simulink model "onolfihjsihjn"  (R2018b)
settings: Solver=FixedStepAuto  StartTime=0.0  StopTime=500  FixedStep=0.1  MaxStep=1E-3  RelTol=1e-3
values from neighbouring files (symbols this model uses):
  Ad = [1  0.1; 0  1]    [data_ver2.mat]    (also in data_ver3.mat = [1  0.5; 0  1]; just_running.m = sysd.A)
  bd = [0.005 0.1]    [data_ver2.mat]    (also in data_ver3.mat = [0.125 0.5]; just_running.m = sysd.B)
  SumoTs = block.DialogPrm(1).Data    [LeaderBlock.m]    (also in ObjectBlock.m; data_ver2.mat = 0.1; data_ver3.mat = 0.5; just_running.m = 0.5)
libraries: simulink x2
settings Model: Creator=HP  LastModifiedBy=HP

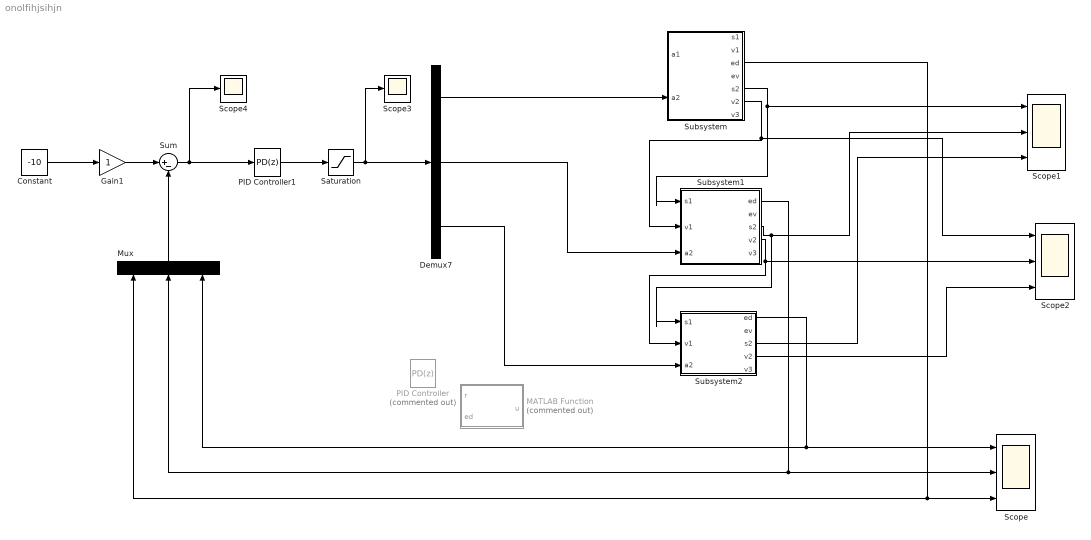
== system onolfihjsihjn ==
  Constant : Constant  Value=-10
  Demux7 : Demux  Outputs=3
  Gain1 : Gain
  MATLAB Function : MATLAB Function  Commented=on  TreatAsAtomicUnit=on
  Mux : Mux  Inputs=3
  PID Controller : simulink/Continuous/PID Controller  Commented=on  Controller=PD  Form=Parallel  TimeDomain=Discrete-time  SampleTime=-1  IntegratorMethod=Forward Euler  FilterMethod=Forward Euler  ControllerParametersSource=internal  P=0.1  I=1  D=1  UseFilter=off  N=1  TunerSelectOption=Transfer Function Based (PID Tuner App)  InitialConditionSource=internal  InitialConditionForIntegrator=0  InitialConditionForFilter=0  DifferentiatorICPrevScaledInput=0  ExternalReset=none  TrackingMode=off  Kt=1  LimitOutput=off  UpperSaturationLimit=inf  LowerSaturationLimit=-inf  LinearizeAsGain=on  AntiWindupMode=none  Kb=1  POutMin=[]  POutMax=[]  IOutMin=[]  IOutMax=[]  DOutMin=[]  DOutMax=[]  NOutMin=[]  NOutMax=[]  SumOutMin=[]  SumOutMax=[]  SaturationOutMin=[]  SaturationOutMax=[]  PParamMin=[]  PParamMax=[]  IParamMin=[]  IParamMax=[]  DParamMin=[]  DParamMax=[]  NParamMin=[]  NParamMax=[]  KbParamMin=[]  KbParamMax=[]  KtParamMin=[]  KtParamMax=[]  KbOutMin=[]  KbOutMax=[]  KtOutMin=[]  KtOutMax=[]  IntegratorOutMin=[]  IntegratorOutMax=[]  FilterOutMin=[]  FilterOutMax=[]  SumI1OutMin=[]  SumI1OutMax=[]  SumI2OutMin=[]  SumI2OutMax=[]  SumI3OutMin=[]  SumI3OutMax=[]  SumI4OutMin=[]  SumI4OutMax=[]  SumDOutMin=[]  SumDOutMax=[]  DifferentiatorOutMin=[]  DifferentiatorOutMax=[]  FilterDiffOutCoefMin=[]  FilterDiffOutCoefMax=[]  ReciprocalOutMin=[]  ReciprocalOutMax=[]  SumDenOutMin=[]  SumDenOutMax=[]  SumNumOutMin=[]  SumNumOutMax=[]  DivideOutMin=[]  DivideOutMax=[]  IntegratorContinuousStateAttributes=''  IntegratorStateMustResolveToSignalObject=off  IntegratorRTWStateStorageClass=Auto  FilterContinuousStateAttributes=''  FilterStateMustResolveToSignalObject=off  FilterRTWStateStorageClass=Auto  ParallelPVariant=InternalParameters  IdealPVariant=Disabled  IVariant=Disabled  DVariant=InternalParameters  IntegratorVariant=Disabled  SatVariant=Disabled  AWVariant=Disabled  PCopyVariant=Disabled  TRVariant=Disabled  FdbkBlocksVariant=Forward  IdealPFdbkVariant=Disabled  SatFdbkVariant=Disabled  DerivativeFilterVariant=Differentiator  NVariant=Passthrough  NCopyVariant=Disabled_SignalSpec  FilterICVariant=InternalICsDifferentiator  IntegratorICVariant=Disabled  ExternalResetVariant=Disabled  TRSumVariant=Passthrough  SumFdbkVariant=Disabled  SumVariant=Sum_PD
  PID Controller1 : simulink/Continuous/PID Controller  Controller=PD  Form=Parallel  TimeDomain=Discrete-time  SampleTime=-1  IntegratorMethod=Forward Euler  FilterMethod=Forward Euler  ControllerParametersSource=internal  P=0.1  I=1  D=0.8  UseFilter=off  N=1  TunerSelectOption=Transfer Function Based (PID Tuner App)  InitialConditionSource=internal  InitialConditionForIntegrator=0  InitialConditionForFilter=0  DifferentiatorICPrevScaledInput=0  ExternalReset=none  TrackingMode=off  Kt=1  LimitOutput=off  UpperSaturationLimit=inf  LowerSaturationLimit=-inf  LinearizeAsGain=on  AntiWindupMode=none  Kb=1  POutMin=[]  POutMax=[]  IOutMin=[]  IOutMax=[]  DOutMin=[]  DOutMax=[]  NOutMin=[]  NOutMax=[]  SumOutMin=[]  SumOutMax=[]  SaturationOutMin=[]  SaturationOutMax=[]  PParamMin=[]  PParamMax=[]  IParamMin=[]  IParamMax=[]  DParamMin=[]  DParamMax=[]  NParamMin=[]  NParamMax=[]  KbParamMin=[]  KbParamMax=[]  KtParamMin=[]  KtParamMax=[]  KbOutMin=[]  KbOutMax=[]  KtOutMin=[]  KtOutMax=[]  IntegratorOutMin=[]  IntegratorOutMax=[]  FilterOutMin=[]  FilterOutMax=[]  SumI1OutMin=[]  SumI1OutMax=[]  SumI2OutMin=[]  SumI2OutMax=[]  SumI3OutMin=[]  SumI3OutMax=[]  SumI4OutMin=[]  SumI4OutMax=[]  SumDOutMin=[]  SumDOutMax=[]  DifferentiatorOutMin=[]  DifferentiatorOutMax=[]  FilterDiffOutCoefMin=[]  FilterDiffOutCoefMax=[]  ReciprocalOutMin=[]  ReciprocalOutMax=[]  SumDenOutMin=[]  SumDenOutMax=[]  SumNumOutMin=[]  SumNumOutMax=[]  DivideOutMin=[]  DivideOutMax=[]  IntegratorContinuousStateAttributes=''  IntegratorStateMustResolveToSignalObject=off  IntegratorRTWStateStorageClass=Auto  FilterContinuousStateAttributes=''  FilterStateMustResolveToSignalObject=off  FilterRTWStateStorageClass=Auto  ParallelPVariant=InternalParameters  IdealPVariant=Disabled  IVariant=Disabled  DVariant=InternalParameters  IntegratorVariant=Disabled  SatVariant=Disabled  AWVariant=Disabled  PCopyVariant=Disabled  TRVariant=Disabled  FdbkBlocksVariant=Forward  IdealPFdbkVariant=Disabled  SatFdbkVariant=Disabled  DerivativeFilterVariant=Differentiator  NVariant=Passthrough  NCopyVariant=Disabled_SignalSpec  FilterICVariant=InternalICsDifferentiator  IntegratorICVariant=Disabled  ExternalResetVariant=Disabled  TRSumVariant=Passthrough  SumFdbkVariant=Disabled  SumVariant=Sum_PD
  Saturation : Saturate  UpperLimit=3  LowerLimit=-5
  Scope : Scope  NumInputPorts=3
  Scope1 : Scope  NumInputPorts=3
  Scope2 : Scope  NumInputPorts=3
  Scope3 : Scope
  Scope4 : Scope
  Subsystem : Subsystem
  Subsystem1 : Subsystem
  Subsystem2 : Subsystem
  Sum : Sum  Inputs=|+-
  wires:
  Constant/1 -> Gain1/1
  Sum/1 -> PID Controller1/1, Scope4/1
  Saturation/1 -> Scope3/1, Demux7/1
  Demux7/1 -> Subsystem/2(a2)
  Demux7/2 -> Subsystem1/3(a2)
  Subsystem/5(s2) -> Subsystem1/1(s1), Scope1/1
  Subsystem/6(v2) -> Scope2/1, Subsystem1/2(v1)
  Subsystem1/3(s2) -> Subsystem2/1(s1), Scope1/2
  Subsystem1/4(v2) -> Subsystem2/2(v1), Scope2/2
  Demux7/3 -> Subsystem2/3(a2)
  Subsystem/3(ed) -> Scope/3, Mux/1
  Subsystem1/1(ed) -> Scope/2, Mux/2
  Subsystem2/1(ed) -> Scope/1, Mux/3
  Subsystem2/3(s2) -> Scope1/3
  Subsystem2/4(v2) -> Scope2/3
  Gain1/1 -> Sum/1
  Mux/1 -> Sum/2
  PID Controller1/1 -> Saturation/1

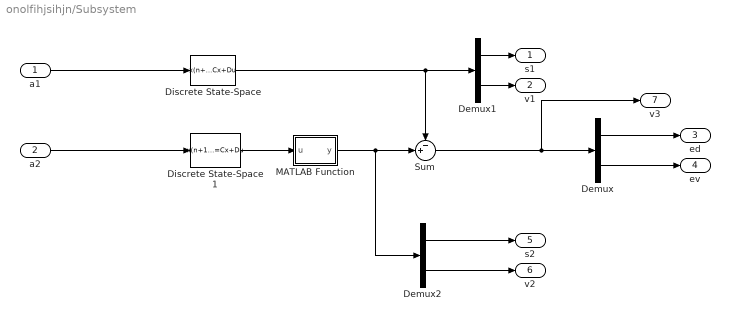
== system onolfihjsihjn/Subsystem ==
  a1 : Inport
  a2 : Inport  Port=2
  Demux : Demux  Outputs=2
  Demux1 : Demux  Outputs=2
  Demux2 : Demux  Outputs=2
  Discrete State-Space : DiscreteStateSpace  A=Ad  B=bd  C=eye(2)  D=zeros(2,1)  InitialCondition=[0;19]  SampleTime=SumoTs
  Discrete State-Space1 : DiscreteStateSpace  A=Ad  B=bd  C=eye(2)  D=zeros(2,1)  InitialCondition=[-100;22]  SampleTime=SumoTs
  MATLAB Function : MATLAB Function  TreatAsAtomicUnit=on
  Sum : Sum  Inputs=-+|
  s1 : Outport
  v1 : Outport  Port=2
  ed : Outport  Port=3
  ev : Outport  Port=4
  s2 : Outport  Port=5
  v2 : Outport  Port=6
  v3 : Outport  Port=7
  wires:
  MATLAB Function/1(y) -> Demux2/1, Sum/2
  Discrete State-Space/1 -> Demux1/1, Sum/1
  Discrete State-Space1/1 -> MATLAB Function/1(u)
  a1/1 -> Discrete State-Space/1
  a2/1 -> Discrete State-Space1/1
  Sum/1 -> v3/1, Demux/1
  Demux/1 -> ed/1
  Demux/2 -> ev/1
  Demux1/1 -> s1/1
  Demux1/2 -> v1/1
  Demux2/1 -> s2/1
  Demux2/2 -> v2/1

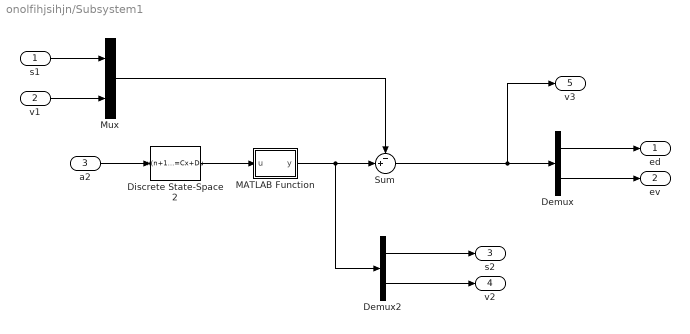
== system onolfihjsihjn/Subsystem1 ==
  s1 : Inport
  v1 : Inport  Port=2
  a2 : Inport  Port=3
  Demux : Demux  Outputs=2
  Demux2 : Demux  Outputs=2
  Discrete State-Space2 : DiscreteStateSpace  A=Ad  B=bd  C=eye(2)  D=zeros(2,1)  InitialCondition=[-200;19]  SampleTime=SumoTs
  MATLAB Function : MATLAB Function  TreatAsAtomicUnit=on
  Mux : Mux  Inputs=2
  Sum : Sum  Inputs=-+|
  ed : Outport
  ev : Outport  Port=2
  s2 : Outport  Port=3
  v2 : Outport  Port=4
  v3 : Outport  Port=5
  wires:
  MATLAB Function/1(y) -> Demux2/1, Sum/2
  Discrete State-Space2/1 -> MATLAB Function/1(u)
  Sum/1 -> v3/1, Demux/1
  Demux/1 -> ed/1
  Demux/2 -> ev/1
  Demux2/1 -> s2/1
  Demux2/2 -> v2/1
  s1/1 -> Mux/1
  v1/1 -> Mux/2
  Mux/1 -> Sum/1
  a2/1 -> Discrete State-Space2/1

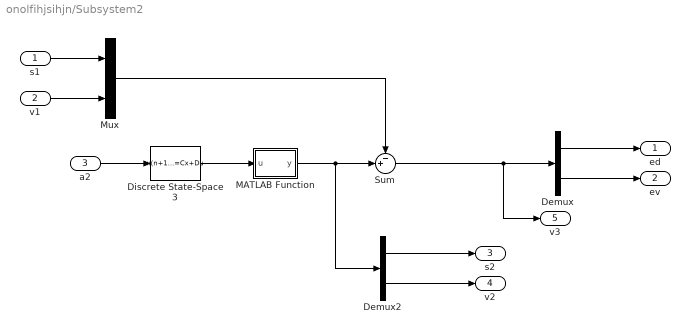
== system onolfihjsihjn/Subsystem2 ==
  s1 : Inport
  v1 : Inport  Port=2
  a2 : Inport  Port=3
  Demux : Demux  Outputs=2
  Demux2 : Demux  Outputs=2
  Discrete State-Space3 : DiscreteStateSpace  A=Ad  B=bd  C=eye(2)  D=zeros(2,1)  InitialCondition=[-280;22]  SampleTime=SumoTs
  MATLAB Function : MATLAB Function  TreatAsAtomicUnit=on
  Mux : Mux  Inputs=2
  Sum : Sum  Inputs=-+|
  ed : Outport
  ev : Outport  Port=2
  s2 : Outport  Port=3
  v2 : Outport  Port=4
  v3 : Outport  Port=5
  wires:
  MATLAB Function/1(y) -> Demux2/1, Sum/2
  Discrete State-Space3/1 -> MATLAB Function/1(u)
  Sum/1 -> v3/1, Demux/1
  Demux/1 -> ed/1
  Demux/2 -> ev/1
  Demux2/1 -> s2/1
  Demux2/2 -> v2/1
  s1/1 -> Mux/1
  v1/1 -> Mux/2
  Mux/1 -> Sum/1
  a2/1 -> Discrete State-Space3/1

== matlab function onolfihjsihjn/Subsystem1/MATLAB Function ==
  data: u input; y output
function y = fcn(u)
if u(2) >= 23
    y = [u(1);23];
elseif u(2) <= 15
    y = [u(1);15];
else
    y = [u(1);u(2)];
end

== matlab function onolfihjsihjn/Subsystem2/MATLAB Function ==
  data: u input; y output
function y = fcn(u)
if u(2) >= 23
    y = [u(1);23];
elseif u(2) <= 15
    y = [u(1);15];
else
    y = [u(1);u(2)];
end

== matlab function onolfihjsihjn/MATLAB Function ==
  data: r input; ed input; u output
function u = fcn(r,ed)
Ts = 0.1;
persistent temp;
if isempty(temp)
    temp = zeros(size(ed));
end

if length(temp) < length(ed)
    temp = [temp;0];
elseif length(temp) > length(ed)
    temp = temp(1:end-1);
end

e0 = r-temp;
e1 = r-ed;

kp = 0.1;
kd = 1;
% u = kp*e1 + kd*(e1-e0)/Ts;
u = kp*e1 + kd*(e1-e0)/Ts;
temp(:) = ed;

== matlab function onolfihjsihjn/Subsystem/MATLAB Function ==
  data: u input; y output
function y = fcn(u)
if u(2) >= 23
    y = [u(1);23];
elseif u(2) <= 15
    y = [u(1);15];
else
    y = [u(1);u(2)];
end
